simulink model "BMS_test_SOC_SOH_multi_cell"  (R2024a)
settings: Solver=FixedStepAuto  StartTime=0.0  StopTime=BMS_time0(end)  FixedStep=.1  RelTol=1e-3
settings Model: DataDictionary=SOXDictionary.sldd  SimulationMode=accelerator  PacingRate=100  Creator=mmackenzie  LastModifiedBy=mmackenzie
settings OptimizationCC: DefaultUnderspecifiedDataType=single
settings DebuggingCC: ParamPrecisionLossAbsoluteDiffThreshold=1e-7  ParamPrecisionLossRelativeDiffThreshold=1e-4  AllowSymbolicDim=off

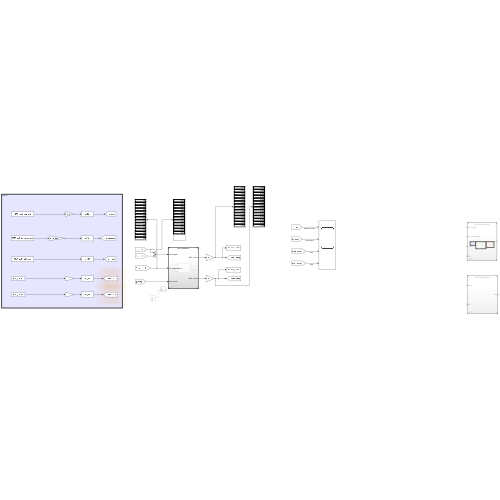
[thumbnail: Simulink's stored preview of the top-level diagram]
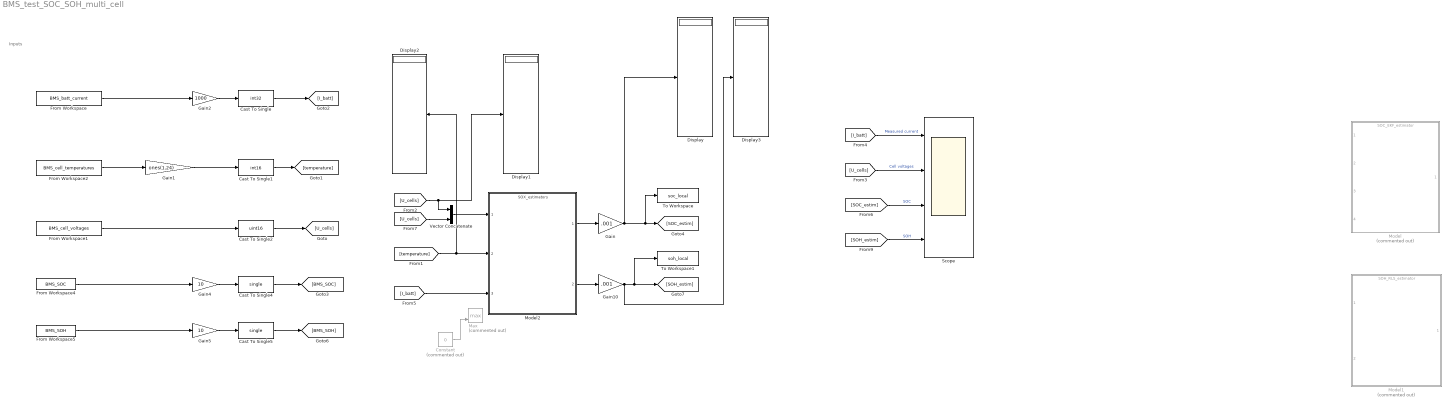
== system BMS_test_SOC_SOH_multi_cell ==
  note: Inputs
  Cast To Single : DataTypeConversion  OutDataTypeStr=int32  SaturateOnIntegerOverflow=off  RndMeth=Floor
  Cast To Single1 : DataTypeConversion  OutDataTypeStr=int16  SaturateOnIntegerOverflow=off  RndMeth=Floor
  Cast To Single2 : DataTypeConversion  OutDataTypeStr=uint16  SaturateOnIntegerOverflow=off  RndMeth=Floor
  Cast To Single4 : DataTypeConversion  OutDataTypeStr=single  SaturateOnIntegerOverflow=off  RndMeth=Floor
  Cast To Single5 : DataTypeConversion  OutDataTypeStr=single  SaturateOnIntegerOverflow=off  RndMeth=Floor
  Constant : Constant  Commented=on  Value=0  OutDataTypeStr=single
  Display{,1..3} (4 alike) : Display
  From Workspace : FromWorkspace  VariableName=BMS_batt_current  SampleTime=-1
  From Workspace1 : FromWorkspace  VariableName=BMS_cell_voltages  SampleTime=-1
  From Workspace2 : FromWorkspace  VariableName=BMS_cell_temperatures  SampleTime=-1
  From Workspace4 : FromWorkspace  VariableName=BMS_SOC  SampleTime=-1
  From Workspace5 : FromWorkspace  VariableName=BMS_SOH  SampleTime=-1
  Gain : Gain  Gain=.001
  Gain1 : Gain  Gain=ones(1,24)
  Gain10 : Gain  Gain=.001
  Gain2 : Gain  Gain=1000
  Gain4 : Gain  Gain=10
  Gain5 : Gain  Gain=10
  Max : MinMax  Commented=on  Function=max  Inputs=2  OutDataTypeStr=single
  Model : ModelReference  Commented=on  ModelNameDialog=SOC_EKF_estimator.slx  SimulationMode=Normal  ModelReferenceVersion=1.52
  Model1 : ModelReference  Commented=on  ModelNameDialog=SOH_RLS_estimator.slx  SimulationMode=Normal  ModelReferenceVersion=1.49
  Model2 : ModelReference  ModelNameDialog=SOX_estimators.slx  SimulationMode=Normal  ModelReferenceVersion=1.9
  Scope : Scope  NumInputPorts=4
  To Workspace : ToWorkspace  VariableName=soc_local  SaveFormat=Timeseries  SampleTime=-1
  To Workspace1 : ToWorkspace  VariableName=soh_local  SaveFormat=Timeseries  SampleTime=-1
  Vector Concatenate : Concatenate
  wires:
  [I_batt] -> Scope/1  "Measured current"
  Model2/1 -> Gain/1
  [SOC_estim] -> Scope/3  "SOC"
  From Workspace4/1 -> Gain4/1
  Gain/1 -> Display/1, To Workspace/1, [SOC_estim]
  From Workspace/1 -> Gain2/1
  From Workspace1/1 -> Cast To Single2/1
  Gain4/1 -> Cast To Single4/1
  Cast To Single/1 -> [I_batt]
  Cast To Single1/1 -> [temperature]
  Cast To Single2/1 -> [U_cells]
  Cast To Single4/1 -> [BMS_SOC]
  [U_cells] -> Scope/2  "Cell voltages"
  From Workspace2/1 -> Gain1/1
  Gain1/1 -> Cast To Single1/1
  [temperature] -> Display2/1, Model2/2
  Gain2/1 -> Cast To Single/1
  From Workspace5/1 -> Gain5/1
  Cast To Single5/1 -> [BMS_SOH]
  Gain5/1 -> Cast To Single5/1
  Model2/2 -> Gain10/1
  [I_batt] -> Model2/3
  Gain10/1 -> Display3/1, [SOH_estim], To Workspace1/1
  [SOH_estim] -> Scope/4  "SOH"
  Constant/1 -> Max/2
  Vector Concatenate/1 -> Model2/1
  [U_cells] -> Display1/1, Vector Concatenate/1
  [U_cells] -> Vector Concatenate/2
